simulink model "code_gen"  (Simulink 7.5)
settings: Solver=FixedStepDiscrete  StartTime=0.0  StopTime=10.0  FixedStep=0.001  RelTol=1e-3
InitFcn:
  | boat_constants
values from neighbouring files (symbols this model uses):
  InitialPoint = 0    [boat_constants.m]    (also in l2plus.m)
  IPStar = 0    [boat_constants.m]    (also in l2plus.m)
  ISA_g = 9.815    [boat_constants.m]
  MaxDwnPthStar = 1    [boat_constants.m]    (also in l2plus.m)
  OC2max = 49999    [boat_constants.m]    (also in simulation_constants.m)
  switchDistance = 4    [boat_constants.m]    (also in l2plus.m)
  T_step = 0.01    [boat_constants.m]    (also in common.m)
  tanIntercept = tan( 45*pi/180 )    [boat_constants.m]    (also in l2plus.m)
  TStar = single(4.5)    [boat_constants.m]    (also in l2plus.m = single(2))
  Turn2Track = 0    [boat_constants.m]    (also in l2plus.m)
undefined symbols (not defined in the file or in its folder): buildAndCheckMessage, buildAndCheckSentence, DiscIntNeverNeededParam, ecan1_buffered_transmit_matlab, ecan1_init, getGpsMainData, getSensorData, u1, y1
libraries: simulink x49, dsPICdrivers x22, simulink_need_slupdate x6, microSimulink x4, aerolibconvert2 x3
(part 2 of 3)

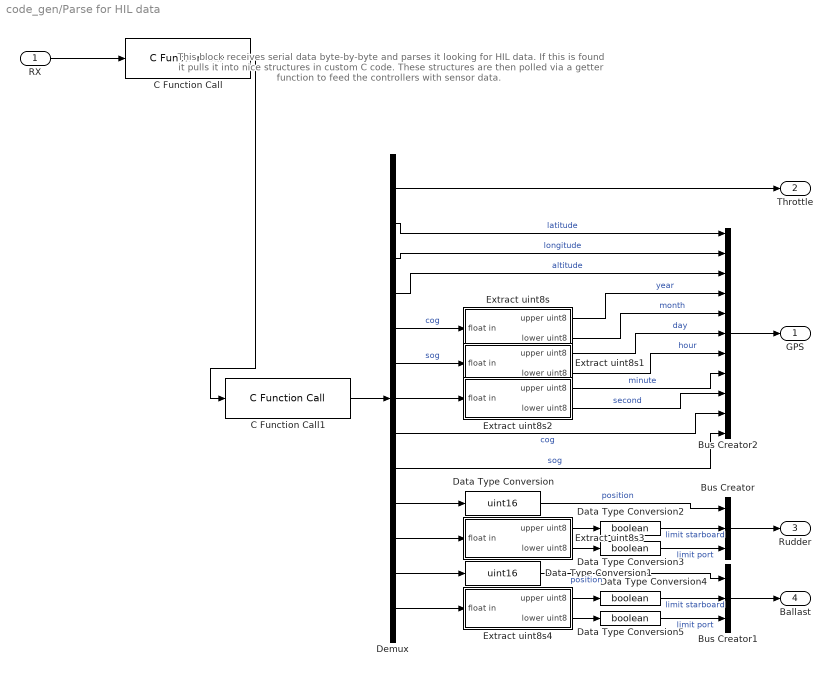
== system code_gen/Parse for HIL data ==
  note: This block receives serial data byte-by-byte and parses it looking for HIL data.
      | If this is found it pulls it into nice structures in custom C code. These structures
      | are then polled via a getter function to feed the controllers with sensor data.
  RX : Inport
  Bus Creator : BusCreator  Inputs=3
  Bus Creator1 : BusCreator  Inputs=3
  Bus Creator2 : BusCreator  Inputs=11
  C Function Call : dsPICdrivers/OTHERS/C Function Call  Tag=dsPIC_dsPIC_CFunctionCall  fctName='buildAndCheckMessage'  INPUT_SIZE=1  INPUT1=uint8  INPUT2=--  INPUT3=--  OUTPUT_SIZE=1  OUTPUT1=--  SampleTime=-1  InputType=[ 2 ]  OutputType=[ ]  FctDeclaration=extern void buildAndCheckMessage(uint8_T u1);  FctCall=buildAndCheckMessage(%u1);  OrderingInOutPopup=Output
  C Function Call1 : dsPICdrivers/OTHERS/C Function Call  Tag=dsPIC_dsPIC_CFunctionCall  fctName='getSensorData'  INPUT_SIZE=1  INPUT1=--  INPUT2=--  INPUT3=--  OUTPUT_SIZE=13  OUTPUT1=real32  SampleTime=.01  InputType=[ ]  OutputType=[ 7 ]  FctDeclaration=extern void getSensorData(real32_T* y1);  FctCall=getSensorData(*%y1);  OrderingInOutPopup=Input
  Data Type Conversion : DataTypeConversion  OutDataTypeMode=uint16  OutDataType=fixdt(1, 16)  OutScaling=2^0  OutDataTypeStr=uint16  ConvertRealWorld=Stored Integer (SI)  RndMeth=Simplest
  Data Type Conversion1 : DataTypeConversion  OutDataTypeMode=uint16  OutDataType=fixdt(1, 16)  OutScaling=2^0  OutDataTypeStr=uint16  ConvertRealWorld=Stored Integer (SI)  RndMeth=Simplest
  Data Type Conversion{2..5} (4 alike) : DataTypeConversion  OutDataTypeMode=boolean  OutDataType=fixdt(1, 16)  OutScaling=2^0  OutDataTypeStr=boolean
  Demux : Demux  Outputs=13
  Extract uint8s : Subsystem
  Extract uint8s1 : Subsystem
  Extract uint8s2 : Subsystem
  Extract uint8s3 : Subsystem
  Extract uint8s4 : Subsystem
  GPS : Outport
  Throttle : Outport  Port=2
  Rudder : Outport  Port=3
  Ballast : Outport  Port=4
  wires:
  RX/1 -> C Function Call/1
  Demux/1 -> Throttle/1
  Bus Creator/1 -> Rudder/1
  Extract uint8s3/1(upper uint8) -> Data Type Conversion2/1
  Demux/10 -> Data Type Conversion/1
  Extract uint8s3/2(lower uint8) -> Data Type Conversion3/1
  Bus Creator1/1 -> Ballast/1
  Extract uint8s4/1(upper uint8) -> Data Type Conversion4/1
  Demux/12 -> Data Type Conversion1/1
  Extract uint8s4/2(lower uint8) -> Data Type Conversion5/1
  Bus Creator2/1 -> GPS/1
  Demux/4 -> Bus Creator2/3  "altitude"
  Demux/3 -> Bus Creator2/2  "longitude"
  Demux/2 -> Bus Creator2/1  "latitude"
  C Function Call1/1 -> Demux/1
  Demux/11 -> Extract uint8s3/1(float in)
  Demux/13 -> Extract uint8s4/1(float in)
  Data Type Conversion/1 -> Bus Creator/1  "position"
  Data Type Conversion1/1 -> Bus Creator1/1  "position"
  Extract uint8s2/2(lower uint8) -> Bus Creator2/9  "second"
  Extract uint8s2/1(upper uint8) -> Bus Creator2/8  "minute"
  Extract uint8s1/2(lower uint8) -> Bus Creator2/7  "hour"
  Extract uint8s1/1(upper uint8) -> Bus Creator2/6  "day"
  Extract uint8s/2(lower uint8) -> Bus Creator2/5  "month"
  Extract uint8s/1(upper uint8) -> Bus Creator2/4  "year"
  Demux/5 -> Extract uint8s/1(float in)  "cog"
  Demux/6 -> Extract uint8s1/1(float in)  "sog"
  Demux/7 -> Extract uint8s2/1(float in)
  Demux/8 -> Bus Creator2/10  "cog"
  Demux/9 -> Bus Creator2/11  "sog"
  Data Type Conversion2/1 -> Bus Creator/2  "limit starboard"
  Data Type Conversion3/1 -> Bus Creator/3  "limit port"
  Data Type Conversion4/1 -> Bus Creator1/2  "limit starboard"
  Data Type Conversion5/1 -> Bus Creator1/3  "limit port"
  C Function Call/1 -> C Function Call1/1

== system code_gen/Propulsion Outputs ==
  note: Propulsion is controlled here via a CAN interface to the motor driver board.
      | ECAN1 is used and several possible commands are transmitted: enable, disable,
      | or change speed, with speed being between -1023 and 1023 taken as a fraction
      | of total speed (1023).
  In1 : Inport  OutDataType=fixdt(1, 16)  OutScaling=2^0
  Bus Selector : BusSelector  OutputSignals=identifier,data,size,trigger
  To Drive Motor : Subsystem  mask(Send ECAN Message){buffer=0, identifier=hex2dec('401'), identifier_from_input=on, ide=off, remote=off, data=[hex2dec('11') hex2dec('12') hex2dec('13') hex2dec('14')], data_length=4, data_from_input=on, c_func_sample_time=.01, trigger_on_input=on}
      mask prompts: identifier_from_input "Identifier from input"; data_length "Data length"; data_from_input "Data from input"; c_func_sample_time "Sample time"; trigger_on_input "Trigger on input"
      mask help: This block allows for the transmission of a message over the ECAN module.
      mask CallbackString:
      | ||mEnables = get_param(gcb,'MaskEnables');
      | enabled = get_param(gcb, 'identifier_from_input');
      | if strcmp(enabled,'on');
      |     replace_block([gcb '/identifier'],'Constant','Inport','noprompt');
      |     mEnables{2} = 'off';
      |     set_param([gcb '/identifier'],'Port','1');
      | else
      |     replace_block([gcb '/identifier'],'Inport','Constant','noprompt');
      |     mEnables{2} = 'on';
      |     set_param([gcb '/identifier'],'Value','identifier');
      | end
      | set_param(gcb, 'MaskEnables', mEnables);
      | |||data = eval(get_param(gcb, 'data'));
      | y = size(data,1);
      | x = size(data,2);
      | if y > 1 && x > 1
      |     error('Data must be a 1-dimensional vector')
      | else
      |     if or(x > 8, y > 8)
      |         error('Data cannot be larger than 8-bytes');
      |     end
      | end
      | 
      | set_param(gcb, 'data_length', num2str(length(data)));|data_length = eval(get_param(gcb, 'data_length'));
      | if or(data_length < 0, data_length > 9)
      |     error('Data cannot be more than 8 bytes or less than 0.')
      | end|mEnables = get_param(gcb,'MaskEnables');
      | enabled = get_param(gcb, 'data_from_input');
      | if strcmp(enabled,'on');
      |     replace_block([gcb '/data'],'Constant','Inport','noprompt');
      |     replace_block([gcb '/data_length'],'Constant','Inport','noprompt');
      |     mEnables{6} = 'off';
      |     mEnables{7} = 'off';
      |     port = 1;
      |     if ~isempty(find_system(gcb,'LookUnderMasks','all','Name','identifier'))
      |         port = 2;
      |     end
      |     set_param([gcb '/data'],'Port',num2str(port));
      |     set_param([gcb '/data_length'],'Port',num2str(port+1));
      | else
      |     replace_block([gcb '/data'],'Inport','Constant','noprompt');
      |     replace_block([gcb '/data_length'],'Inport','Constant','noprompt');
      |     mEnables{6} = 'on';
      |     mEnables{7} = 'on';
      |     set_param([gcb '/data'],'Value','data');
      |     set_param([gcb '/data'],'OutDataTypeMode','uint8');
      |     set_param([gcb '/data_length'],'Value','data_length');
      |     set_param([gcb '/data_length'],'OutDataTypeMode','uint8');
      | end
      | set_param(gcb, 'MaskEnables', mEnables);
      | ||mEnables = get_param(gcb,'MaskEnables');
      | enabled = get_param(gcb, 'trigger_on_input');
      | c_func_blk = find_system(gcb,'LookUnderMasks','all','FunctionName','dsPIC_C_function_Call');
      | if strcmp(enabled,'on');
      |     mEnables{9} = 'off';
      |     %set_param(c_func_blk,'SampleTime','-1');
      |     replace_block([gcb '/trigger'],'Constant','Inport','noprompt');
      | else
      |     mEnables{9} = 'on';
      |     %set_param(c_func_blk,'SampleTime','c_func_sample_time');
      |     replace_block([gcb '/trigger'],'Inport','Constant','noprompt');
      |     %set_param([gcb '/trigger'],'Value','1');
      | end
      | set_param(gcb, 'MaskEnables', mEnables);
      mask Display: disp('ECAN1 TX');
  wires:
  In1/1 -> Bus Selector/1
  Bus Selector/1 -> To Drive Motor/1(identifier)  "<identifier>"
  Bus Selector/2 -> To Drive Motor/2(data)  "<data>"
  Bus Selector/3 -> To Drive Motor/3(data_length)  "<size>"
  Bus Selector/4 -> To Drive Motor/4(trigger)  "<trigger>"

== system code_gen/Radio Control Inputs ==
  note: IC2 is used to control the reset as the throttle has a heartbeat PWM output upon disconnect.
      | Every other channel will be disabled with no pulses, so anything besides the throttle channel
      | should work fine.
  Clear to Zero if Disconnect : Subsystem
  Compare To Constant : simulink/Logic and Bit Operations/Compare To Constant  SystemSampleTime=-1  relop=>  const=7500  LogicOutDataTypeMode=boolean
  RC Input : dsPICdrivers/Peripheral I//O/Input Capture  Tag=dsPIC_PWM_IC  Priority=5  IntPriority=7  Channel=[2 3 4]  Channel_UP_Down_Periode="[1  1  1]"  MaxChannel="[0.002       0.002       0.002]"  SafeMarge="[10  10  10]"  MaxName=' IC2max , IC3max , IC4max '  Precision="[13.425       13.425       13.425]"  Timer="[2  2  2]"  ChangeDetected="[2  2  2]"  ChangeDetectedPortRef=3  SampleTime=.1  Status=OK
  Rate Transition : RateTransition
  Rate Transition1 : RateTransition
  Rate Transition2 : RateTransition
  Terminator1 : Terminator
  Terminator2 : Terminator
  Rudder : Outport
  Throttle : Outport  Port=2
  Mode : Outport  Port=3
  wires:
  Clear to Zero if Disconnect/2(o2) -> Rate Transition1/1
  Clear to Zero if Disconnect/1(o1) -> Rate Transition/1
  Clear to Zero if Disconnect/3(o3) -> Rate Transition2/1
  RC Input/1 -> Clear to Zero if Disconnect/2(ch1)
  RC Input/3 -> Clear to Zero if Disconnect/3(ch2)
  RC Input/5 -> Clear to Zero if Disconnect/4(ch3)
  Rate Transition/1 -> Rudder/1
  Rate Transition1/1 -> Throttle/1
  Rate Transition2/1 -> Compare To Constant/1
  RC Input/2 -> Clear to Zero if Disconnect/1(Reset)
  RC Input/6 -> Terminator1/1
  Compare To Constant/1 -> Mode/1
  RC Input/4 -> Terminator2/1

== system code_gen/Rudder Outputs ==
  note: Rudder commands are output via a pulse-train signaling step (through the OC2 pins),
      | a direction bit set via RD5, and an enable bit set via RG9.
  In1 : Inport
  Bus Selector : BusSelector  OutputSignals=enable,direction,up,period
  Digital Output Write : dsPICdrivers/Digital I//O/Digital Output Write  Tag=dsPIC_Digital_Output  Priority=5  PORT=D  Pin=[5]  Simultaneous=off  OrderingInOutPopup=None
  Digital Output Write1 : dsPICdrivers/Digital I//O/Digital Output Write  Tag=dsPIC_Digital_Output  Priority=5  PORT=G  Pin=[9]  Simultaneous=off  OrderingInOutPopup=None
  Rudder Motor : dsPICdrivers/Peripheral I//O/Output Compare  Tag=dsPIC_PWM_out  Priority=5  IntPriority=3  CHANNEL=[2]  Channel_UP_Down_Periode=[5]  MaxChannel=[0.01]  MaxName=' OC2max '  Precision=[15.6096]  Timer=[2]  Status=OK  SafeMarge=[0]  PortLetter=[68]  PortNumber=[1]  MaxValues=[49999]
  wires:
  Bus Selector/2 -> Digital Output Write/1  "<direction>"
  Bus Selector/1 -> Digital Output Write1/1  "<enable>"
  Bus Selector/3 -> Rudder Motor/1  "<up>"
  Bus Selector/4 -> Rudder Motor/2  "<period>"
  In1/1 -> Bus Selector/1

== system code_gen/Rudder Sensors ==
  note: The rudder has two main sensors: hall effect and a potentiometer. The
      | potentiometer returns a voltage value through the onboard ADC indicating
      | rudder position exactly. The three Hall effect sensors are used as limit switches
      | indicating port and starboard limits as well as center, though this sensor isn't
      | being used currently.
      |
      | It expects a range of 1.12-2.11V for the rudder position potentiometer with
      | 2.11V being hard to port. The potentiometer was powered at 3.3V for these
      | measurements.
  Bus Creator : BusCreator  Inputs=3
  Port Hall : dsPICdrivers/Digital I//O/Digital Input  Tag=dsPIC_Digital_Input  PORT=F  Pin=[3]  SampleTime=.01  OrderingInOutPopup=None
  Rudder Potentiometer : dsPICdrivers/Peripheral I//O/ADC Input  Tag=dsPIC_ADC  Priority=5  ADC_TYPE=10 bits  ADC_MODE=Continuous sampling & get last channel value  NbrSampleStep=1  VoltRefpopup="AVdd  -  AVss"  OutFormatBitspopup=ssss sssd dddd dddd : Signed Integer  InterruptPriority=6  ANCHANNELS=[0]  MaxName=ANmax = 1023  Rin=1e2  ADCS=12  SAMC=1  Temperature=25  DMAChannel=7  SampleTime=.01  Status="OK  |  Tsmp=1.625e-007 |  T/Channel=2.113e-006 |  Tall=2.113e-006"  SSRC=auto convert
  Starboard Hall : dsPICdrivers/Digital I//O/Digital Input  Tag=dsPIC_Digital_Input  PORT=G  Pin=[3]  SampleTime=.01  OrderingInOutPopup=None
  Out1 : Outport
  wires:
  Rudder Potentiometer/1 -> Bus Creator/1  "position"
  Starboard Hall/1 -> Bus Creator/2  "limit starboard"
  Port Hall/1 -> Bus Creator/3  "limit port"
  Bus Creator/1 -> Out1/1

== system code_gen/Throttle Command ==
  sensors : Inport
  speed : Inport  Port=2
  Bus Creator : BusCreator
  Mux Everything : Subsystem
  Terminator : Terminator
  Trigger Events : Subsystem
  command : Outport  OutDataType=sfix(16)  OutScaling=2^0
  wires:
  sensors/1 -> Terminator/1
  Bus Creator/1 -> command/1
  Trigger Events/1(Change Speed) -> Mux Everything/1(speed)
  Trigger Events/3(Enable) -> Mux Everything/3(enable)
  Trigger Events/2(Disable) -> Mux Everything/2(disable)
  speed/1 -> Mux Everything/4(Throttle), Trigger Events/1(RC Throttle)
  Mux Everything/1(iden) -> Bus Creator/1  "identifier"
  Mux Everything/2(data) -> Bus Creator/2  "data"
  Mux Everything/3(size) -> Bus Creator/3  "size"
  Mux Everything/4(trig) -> Bus Creator/4  "trigger"

== system code_gen/Throttle Sensors ==
  note: Throttle output is currently being ignored. The motor driver board
      | should report current velocity along with other status information
      | on a regular basis and that could be parsed for this information. As
      | of right now it's been deemed non-critical and therefore ignored.
  Constant : Constant  Value=0  OutDataType=fixdt(1, 16)  OutScaling=2^0  SampleTime=.01
  Out1 : Outport
  wires:
  Constant/1 -> Out1/1

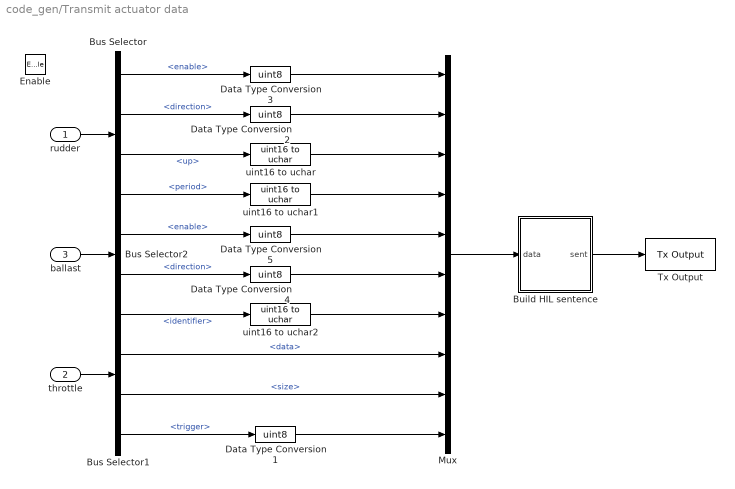
== system code_gen/Transmit actuator data ==
  rudder : Inport  OutDataType=fixdt(1, 16)  OutScaling=2^0
  throttle : Inport  Port=2  OutDataType=fixdt(1, 16)  OutScaling=2^0
  ballast : Inport  Port=3  OutDataType=fixdt(1, 16)  OutScaling=2^0
  Enable : EnablePort
  Build HIL sentence : Subsystem
  Bus Selector : BusSelector  OutputSignals=enable,direction,up,period
  Bus Selector1 : BusSelector  OutputSignals=identifier,data,size,trigger
  Bus Selector2 : BusSelector  OutputSignals=enable,direction
  Data Type Conversion{1..5} (5 alike) : DataTypeConversion  OutDataTypeMode=uint8  OutDataType=fixdt(1, 16)  OutScaling=2^0  OutDataTypeStr=uint8
  Mux : Mux  Inputs=10
  Tx Output : dsPICdrivers/Serial PORT/Tx Output  Tag=dsPIC_TX  Priority=5  UART=2  OrderingInOutPopup=None
  uint16 to uchar : microSimulink/Conversions/uint16 to uchar  SystemSampleTime=-1
  uint16 to uchar1 : microSimulink/Conversions/uint16 to uchar  SystemSampleTime=-1
  uint16 to uchar2 : microSimulink/Conversions/uint16 to uchar  SystemSampleTime=-1
  wires:
  rudder/1 -> Bus Selector/1
  Bus Selector/2 -> Data Type Conversion2/1  "<direction>"
  Bus Selector/1 -> Data Type Conversion3/1  "<enable>"
  throttle/1 -> Bus Selector1/1
  Bus Selector1/4 -> Data Type Conversion1/1  "<trigger>"
  Data Type Conversion2/1 -> Mux/2
  Bus Selector1/3 -> Mux/9  "<size>"
  Bus Selector1/1 -> uint16 to uchar2/1  "<identifier>"
  Data Type Conversion1/1 -> Mux/10
  Build HIL sentence/1(sent) -> Tx Output/1
  Mux/1 -> Build HIL sentence/1(data)
  Data Type Conversion3/1 -> Mux/1
  Bus Selector/3 -> uint16 to uchar/1  "<up>"
  ballast/1 -> Bus Selector2/1
  Bus Selector2/1 -> Data Type Conversion5/1  "<enable>"
  Bus Selector2/2 -> Data Type Conversion4/1  "<direction>"
  Bus Selector/4 -> uint16 to uchar1/1  "<period>"
  uint16 to uchar/1 -> Mux/3
  uint16 to uchar1/1 -> Mux/4
  uint16 to uchar2/1 -> Mux/7
  Bus Selector1/2 -> Mux/8  "<data>"
  Data Type Conversion4/1 -> Mux/6
  Data Type Conversion5/1 -> Mux/5

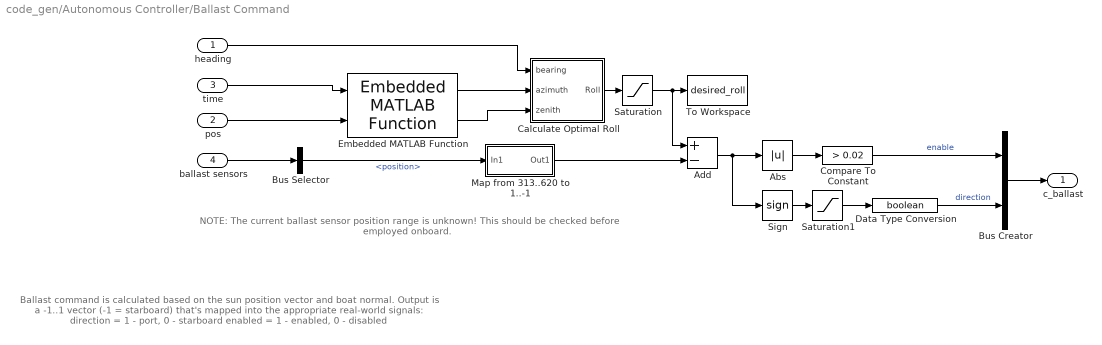
== system code_gen/Autonomous Controller/Ballast Command ==
  note: Ballast command is calculated based on the sun position vector
      | and boat normal. Output is a -1..1 vector (-1 = starboard) that's
      |  mapped into the appropriate real-world signals:
      | direction = 1 - port, 0 - starboard
      | enabled = 1 - enabled, 0 - disabled
  note: NOTE: The current ballast sensor position range is
      | unknown! This should be checked before employed
      | onboard.
  heading : Inport
  pos : Inport  Port=2
  time : Inport  Port=3
  ballast sensors : Inport  Port=4
  Abs : Abs  OutDataType=fixdt(1, 16)  OutScaling=2^0
  Add : Sum  Inputs=+-  OutDataType=fixdt(1, 16)  OutScaling=2^-10
  Bus Creator : BusCreator  Inputs=2
  Bus Selector : BusSelector  OutputSignals=position
  Calculate Optimal Roll : Subsystem
  Compare To Constant : simulink/Logic and Bit Operations/Compare To Constant  SystemSampleTime=-1  relop=>  const=0.02  LogicOutDataTypeMode=boolean
  Data Type Conversion : DataTypeConversion  OutDataTypeMode=boolean  OutDataType=fixdt(1, 16)  OutScaling=2^0  OutDataTypeStr=boolean  RndMeth=Simplest
  Embedded MATLAB Function : microSimulink/Embedded MATLAB Function  SystemSampleTime=-1
  Map from 313..620 to 1..-1 : Subsystem
  Saturation : Saturate  UpperLimit=1  LowerLimit=-1
  Saturation1 : Saturate  UpperLimit=1  LowerLimit=0  OutDataTypeStr=Inherit: Inherit via back propagation
  Sign : Signum
  To Workspace : ToWorkspace  VariableName=desired_roll  SampleTime=-1  SaveFormat=Structure
  c_ballast : Outport
  wires:
  Data Type Conversion/1 -> Bus Creator/2  "direction"
  Calculate Optimal Roll/1(Roll) -> Saturation/1
  time/1 -> Embedded MATLAB Function/1
  Bus Creator/1 -> c_ballast/1
  ballast sensors/1 -> Bus Selector/1
  Bus Selector/1 -> Map from 313..620 to 1..-1/1(In1)  "<position>"
  Saturation/1 -> Add/1, To Workspace/1
  Add/1 -> Abs/1, Sign/1
  Sign/1 -> Saturation1/1
  Abs/1 -> Compare To Constant/1
  Compare To Constant/1 -> Bus Creator/1  "enable"
  Saturation1/1 -> Data Type Conversion/1
  pos/1 -> Embedded MATLAB Function/2
  heading/1 -> Calculate Optimal Roll/1(bearing)
  Embedded MATLAB Function/1 -> Calculate Optimal Roll/2(azimuth)
  Embedded MATLAB Function/2 -> Calculate Optimal Roll/3(zenith)
  Map from 313..620 to 1..-1/1(Out1) -> Add/2

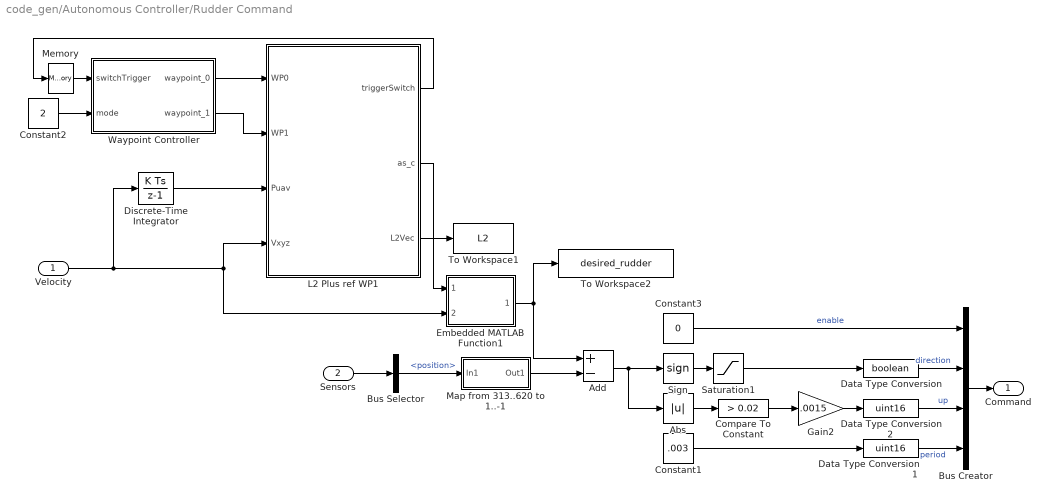
== system code_gen/Autonomous Controller/Rudder Command ==
  Velocity : Inport
  Sensors : Inport  Port=2
  Abs : Abs  OutDataType=fixdt(1, 16)  OutScaling=2^0
  Add : Sum  Inputs=+-  OutDataType=fixdt(1, 16)  OutScaling=2^-10
  Bus Creator : BusCreator
  Bus Selector : BusSelector  OutputSignals=position
  Compare To Constant : simulink/Logic and Bit Operations/Compare To Constant  SystemSampleTime=-1  relop=>  const=0.02  LogicOutDataTypeMode=uint8
  Constant1 : Constant  Value=.003  OutDataTypeMode=single  OutDataType=sfix(16)  OutScaling=2^0  OutDataTypeStr=single
  Constant2 : Constant  Value=2  OutDataTypeMode=uint8  OutDataType=sfix(16)  OutScaling=2^0  OutDataTypeStr=uint8
  Constant3 : Constant  Value=0  OutDataTypeMode=boolean  OutDataType=sfix(16)  OutScaling=2^0  OutDataTypeStr=boolean
  Data Type Conversion : DataTypeConversion  OutDataTypeMode=boolean  OutDataType=fixdt(1, 16)  OutScaling=2^0  OutDataTypeStr=boolean  RndMeth=Simplest
  Data Type Conversion1 : DataTypeConversion  OutDataTypeMode=uint16  OutDataType=fixdt(1, 16)  OutScaling=2^0  OutDataTypeStr=uint16  RndMeth=Simplest
  Data Type Conversion2 : DataTypeConversion  OutDataTypeMode=uint16  OutDataType=fixdt(1, 16)  OutScaling=2^0  OutDataTypeStr=uint16  RndMeth=Simplest
  Discrete-Time Integrator : DiscreteIntegrator  InitialConditionMode=State only (most efficient)  SampleTime=T_step  OutDataType=fixdt(1, 16)  OutScaling=2^0  ICPrevOutput=DiscIntNeverNeededParam  ICPrevScaledInput=DiscIntNeverNeededParam
  Embedded MATLAB Function1 : Stateflow chart  TreatAsAtomicUnit=on
  Gain2 : Gain  Gain=.0015  ParameterDataType=sfix(16)  ParameterScaling=2^0  OutDataTypeMode=single  OutDataType=sfix(16)  OutScaling=2^0  OutDataTypeStr=single
  L2 Plus ref WP1 : Stateflow chart  TreatAsAtomicUnit=on  SystemSampleTime=.01
  Map from 313..620 to 1..-1 : Subsystem
  Memory : Memory  InheritSampleTime=on
  Saturation1 : Saturate  UpperLimit=1  LowerLimit=0  OutDataTypeStr=Inherit: Inherit via back propagation
  Sign : Signum
  To Workspace1 : ToWorkspace  VariableName=L2  SampleTime=-1  SaveFormat=Array
  To Workspace2 : ToWorkspace  VariableName=desired_rudder  SampleTime=-1  SaveFormat=Array
  Waypoint Controller : Stateflow chart  TreatAsAtomicUnit=on
      settings: MinAlgLoopOccurrences=on
  Command : Outport
  wires:
  Constant3/1 -> Bus Creator/1  "enable"
  Data Type Conversion2/1 -> Bus Creator/3  "up"
  Data Type Conversion1/1 -> Bus Creator/4  "period"
  L2 Plus ref WP1/2(as_c) -> Embedded MATLAB Function1/1(lat_accel)
  Velocity/1 -> L2 Plus ref WP1/4(Vxyz), Embedded MATLAB Function1/2(velocity), Discrete-Time Integrator/1
  L2 Plus ref WP1/3(L2Vec) -> To Workspace1/1
  Waypoint Controller/2(waypoint_1) -> L2 Plus ref WP1/2(WP1)
  Waypoint Controller/1(waypoint_0) -> L2 Plus ref WP1/1(WP0)
  L2 Plus ref WP1/1(triggerSwitch) -> Memory/1
  Constant2/1 -> Waypoint Controller/2(mode)
  Memory/1 -> Waypoint Controller/1(switchTrigger)
  Embedded MATLAB Function1/1(rudder) -> To Workspace2/1, Add/1
  Add/1 -> Abs/1, Sign/1
  Sign/1 -> Saturation1/1
  Abs/1 -> Compare To Constant/1
  Compare To Constant/1 -> Gain2/1
  Saturation1/1 -> Data Type Conversion/1
  Gain2/1 -> Data Type Conversion2/1
  Constant1/1 -> Data Type Conversion1/1
  Bus Creator/1 -> Command/1
  Sensors/1 -> Bus Selector/1
  Discrete-Time Integrator/1 -> L2 Plus ref WP1/3(Puav)
  Map from 313..620 to 1..-1/1(Out1) -> Add/2
  Bus Selector/1 -> Map from 313..620 to 1..-1/1(In1)  "<position>"
  Data Type Conversion/1 -> Bus Creator/2  "direction"

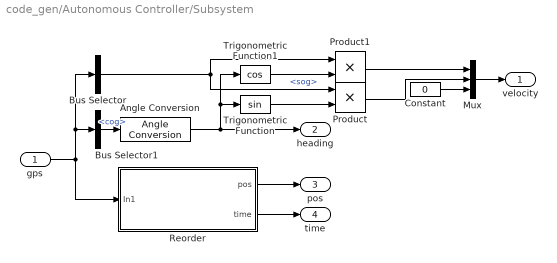
== system code_gen/Autonomous Controller/Subsystem ==
  gps : Inport
  Angle Conversion : aerolibconvert2/Angle Conversion  SystemSampleTime=-1  IU=deg  OU=rad
  Bus Selector : BusSelector  OutputSignals=sog
  Bus Selector1 : BusSelector  OutputSignals=cog
  Constant : Constant  Value=0  OutDataTypeMode=single  OutDataType=fixdt(1, 16)  OutScaling=2^0  OutDataTypeStr=single
  Mux : Mux  Inputs=3
  Product : Product  OutDataTypeMode=single  OutDataType=fixdt(1, 16)  OutScaling=2^0  OutDataTypeStr=single  RndMeth=Zero
  Product1 : Product  OutDataTypeMode=single  OutDataType=fixdt(1, 16)  OutScaling=2^0  OutDataTypeStr=single  RndMeth=Zero
  Reorder : Subsystem
  Trigonometric Function : Trigonometry
  Trigonometric Function1 : Trigonometry  Operator=cos
  velocity : Outport
  heading : Outport  Port=2
  pos : Outport  Port=3
  time : Outport  Port=4
  wires:
  gps/1 -> Bus Selector/1, Bus Selector1/1, Reorder/1(In1)
  Bus Selector1/1 -> Angle Conversion/1  "<cog>"
  Trigonometric Function/1 -> Product/2
  Trigonometric Function1/1 -> Product1/2
  Product1/1 -> Mux/1
  Product/1 -> Mux/2
  Constant/1 -> Mux/3
  Mux/1 -> velocity/1
  Angle Conversion/1 -> heading/1, Trigonometric Function/1, Trigonometric Function1/1
  Bus Selector/1 -> Product1/1, Product/1  "<sog>"
  Reorder/1(pos) -> pos/1
  Reorder/2(time) -> time/1

== system code_gen/Autonomous Controller/Throttle Command ==
  sensors : Inport
  speed : Inport  Port=2
  Bus Creator : BusCreator
  Mux Everything : Subsystem
  Terminator : Terminator
  Trigger Events : Subsystem
  command : Outport  OutDataType=sfix(16)  OutScaling=2^0
  wires:
  Mux Everything/4(trig) -> Bus Creator/4  "trigger"
  Mux Everything/3(size) -> Bus Creator/3  "size"
  Mux Everything/2(data) -> Bus Creator/2  "data"
  Mux Everything/1(iden) -> Bus Creator/1  "identifier"
  speed/1 -> Trigger Events/1(RC Throttle), Mux Everything/4(Throttle)
  Trigger Events/2(Disable) -> Mux Everything/2(disable)
  Trigger Events/3(Enable) -> Mux Everything/3(enable)
  Trigger Events/1(Change Speed) -> Mux Everything/1(speed)
  Bus Creator/1 -> command/1
  sensors/1 -> Terminator/1

== system code_gen/Manual Rudder Command/Map position  into -1024..1023 ==
  input : Inport  OutDataType=sfix(16)  OutScaling=2^0
  Saturation : Saturate  UpperLimit=1023  LowerLimit=-1024
  Weighted Moving Average1 : simulink_need_slupdate/Weighted Moving Average  mgainval=[.5 .5]  vinit=0.0  samptime=-1  OutDataTypeStr=Inherit: Inherit via back propagation  OutDataType=sfix(16)  OutScaling=2^-10  DoSatur=off  GainDataType=uint(16)  MatRadixGroup=Best Precision: Matrix-wise  GainScaling=2^-10
  mapped : Outport  OutDataType=sfix(16)  OutScaling=2^0
  wires:
  Saturation/1 -> Weighted Moving Average1/1
  input/1 -> Saturation/1
  Weighted Moving Average1/1 -> mapped/1

== system code_gen/Manual Rudder Command/Map throttle into -1023..1023 ==
  in : Inport  OutDataType=sfix(16)  OutScaling=2^0
  Bias1 : Bias  Bias=-7215
  Data Type Conversion : DataTypeConversion  OutDataTypeMode=int32  OutDataType=sfix(16)  OutScaling=2^0  OutDataTypeStr=int32
  Data Type Conversion2 : DataTypeConversion  OutDataTypeMode=int16  OutDataType=sfix(16)  OutScaling=2^0  OutDataTypeStr=int16
  Saturation2 : Saturate  UpperLimit=1023  LowerLimit=-1023
  Shift Arithmetic : simulink/Logic and Bit Operations/Shift Arithmetic  SystemSampleTime=-1  nBitShiftRight=10  nBinPtShiftRight=0
  Weighted Moving Average : simulink_need_slupdate/Weighted Moving Average  mgainval=[.2 .2 .2 .2 .2]  vinit=0.0  samptime=-1  OutDataTypeStr=Inherit: Inherit via back propagation  OutDataType=sfix(16)  OutScaling=2^-10  DoSatur=off  GainDataType=uint(16)  MatRadixGroup=Best Precision: Matrix-wise  GainScaling=2^-10
  out : Outport  OutDataType=sfix(16)  OutScaling=2^0
  wires:
  Saturation2/1 -> Weighted Moving Average/1
  Weighted Moving Average/1 -> out/1
  Data Type Conversion2/1 -> Saturation2/1
  Bias1/1 -> Shift Arithmetic/1
  Data Type Conversion/1 -> Bias1/1
  Shift Arithmetic/1 -> Data Type Conversion2/1
  in/1 -> Data Type Conversion/1

== system code_gen/Parse for HIL data/Extract uint8s ==
  float in : Inport
  Data Type Conversion : DataTypeConversion  OutDataTypeMode=uint32  OutDataType=fixdt(1, 16)  OutScaling=2^0  OutDataTypeStr=uint32  ConvertRealWorld=Stored Integer (SI)  RndMeth=Simplest
  Data Type Conversion2 : DataTypeConversion  OutDataTypeMode=uint8  OutDataType=fixdt(1, 16)  OutScaling=2^0  OutDataTypeStr=uint8
  Data Type Conversion3 : DataTypeConversion  OutDataTypeMode=uint8  OutDataType=fixdt(1, 16)  OutScaling=2^0  OutDataTypeStr=uint8
  Extract Bits : simulink/Logic and Bit Operations/Extract Bits  SystemSampleTime=-1  bitsToExtract=Upper half  numBits=8  bitIdxRange=[0 7]  outScalingMode=Treat bit field as an integer
  Extract Bits1 : simulink/Logic and Bit Operations/Extract Bits  SystemSampleTime=-1  bitsToExtract=Lower half  numBits=8  bitIdxRange=[0 7]  outScalingMode=Treat bit field as an integer
  upper uint8 : Outport
  lower uint8 : Outport  Port=2
  wires:
  Data Type Conversion/1 -> Extract Bits/1, Extract Bits1/1
  Extract Bits/1 -> Data Type Conversion2/1
  float in/1 -> Data Type Conversion/1
  Extract Bits1/1 -> Data Type Conversion3/1
  Data Type Conversion2/1 -> upper uint8/1
  Data Type Conversion3/1 -> lower uint8/1

== system code_gen/Parse for HIL data/Extract uint8s1 ==
  float in : Inport
  Data Type Conversion : DataTypeConversion  OutDataTypeMode=uint32  OutDataType=fixdt(1, 16)  OutScaling=2^0  OutDataTypeStr=uint32  ConvertRealWorld=Stored Integer (SI)  RndMeth=Simplest
  Data Type Conversion2 : DataTypeConversion  OutDataTypeMode=uint8  OutDataType=fixdt(1, 16)  OutScaling=2^0  OutDataTypeStr=uint8
  Data Type Conversion3 : DataTypeConversion  OutDataTypeMode=uint8  OutDataType=fixdt(1, 16)  OutScaling=2^0  OutDataTypeStr=uint8
  Extract Bits : simulink/Logic and Bit Operations/Extract Bits  SystemSampleTime=-1  bitsToExtract=Upper half  numBits=8  bitIdxRange=[0 7]  outScalingMode=Treat bit field as an integer
  Extract Bits1 : simulink/Logic and Bit Operations/Extract Bits  SystemSampleTime=-1  bitsToExtract=Lower half  numBits=8  bitIdxRange=[0 7]  outScalingMode=Treat bit field as an integer
  upper uint8 : Outport
  lower uint8 : Outport  Port=2
  wires:
  Data Type Conversion3/1 -> lower uint8/1
  Data Type Conversion2/1 -> upper uint8/1
  Extract Bits1/1 -> Data Type Conversion3/1
  float in/1 -> Data Type Conversion/1
  Extract Bits/1 -> Data Type Conversion2/1
  Data Type Conversion/1 -> Extract Bits1/1, Extract Bits/1

== system code_gen/Parse for HIL data/Extract uint8s2 ==
  float in : Inport
  Data Type Conversion : DataTypeConversion  OutDataTypeMode=uint32  OutDataType=fixdt(1, 16)  OutScaling=2^0  OutDataTypeStr=uint32  ConvertRealWorld=Stored Integer (SI)  RndMeth=Simplest
  Data Type Conversion2 : DataTypeConversion  OutDataTypeMode=uint8  OutDataType=fixdt(1, 16)  OutScaling=2^0  OutDataTypeStr=uint8
  Data Type Conversion3 : DataTypeConversion  OutDataTypeMode=uint8  OutDataType=fixdt(1, 16)  OutScaling=2^0  OutDataTypeStr=uint8
  Extract Bits : simulink/Logic and Bit Operations/Extract Bits  SystemSampleTime=-1  bitsToExtract=Upper half  numBits=8  bitIdxRange=[0 7]  outScalingMode=Treat bit field as an integer
  Extract Bits1 : simulink/Logic and Bit Operations/Extract Bits  SystemSampleTime=-1  bitsToExtract=Lower half  numBits=8  bitIdxRange=[0 7]  outScalingMode=Treat bit field as an integer
  upper uint8 : Outport
  lower uint8 : Outport  Port=2
  wires:
  Data Type Conversion/1 -> Extract Bits/1, Extract Bits1/1
  Extract Bits/1 -> Data Type Conversion2/1
  float in/1 -> Data Type Conversion/1
  Extract Bits1/1 -> Data Type Conversion3/1
  Data Type Conversion2/1 -> upper uint8/1
  Data Type Conversion3/1 -> lower uint8/1

== system code_gen/Parse for HIL data/Extract uint8s3 ==
  float in : Inport
  Data Type Conversion : DataTypeConversion  OutDataTypeMode=uint32  OutDataType=fixdt(1, 16)  OutScaling=2^0  OutDataTypeStr=uint32  ConvertRealWorld=Stored Integer (SI)  RndMeth=Simplest
  Data Type Conversion2 : DataTypeConversion  OutDataTypeMode=uint8  OutDataType=fixdt(1, 16)  OutScaling=2^0  OutDataTypeStr=uint8
  Data Type Conversion3 : DataTypeConversion  OutDataTypeMode=uint8  OutDataType=fixdt(1, 16)  OutScaling=2^0  OutDataTypeStr=uint8
  Extract Bits : simulink/Logic and Bit Operations/Extract Bits  SystemSampleTime=-1  bitsToExtract=Upper half  numBits=8  bitIdxRange=[0 7]  outScalingMode=Treat bit field as an integer
  Extract Bits1 : simulink/Logic and Bit Operations/Extract Bits  SystemSampleTime=-1  bitsToExtract=Lower half  numBits=8  bitIdxRange=[0 7]  outScalingMode=Treat bit field as an integer
  upper uint8 : Outport
  lower uint8 : Outport  Port=2
  wires:
  Data Type Conversion3/1 -> lower uint8/1
  Data Type Conversion2/1 -> upper uint8/1
  Extract Bits1/1 -> Data Type Conversion3/1
  float in/1 -> Data Type Conversion/1
  Extract Bits/1 -> Data Type Conversion2/1
  Data Type Conversion/1 -> Extract Bits1/1, Extract Bits/1

== system code_gen/Parse for HIL data/Extract uint8s4 ==
  float in : Inport
  Data Type Conversion : DataTypeConversion  OutDataTypeMode=uint32  OutDataType=fixdt(1, 16)  OutScaling=2^0  OutDataTypeStr=uint32  ConvertRealWorld=Stored Integer (SI)  RndMeth=Simplest
  Data Type Conversion2 : DataTypeConversion  OutDataTypeMode=uint8  OutDataType=fixdt(1, 16)  OutScaling=2^0  OutDataTypeStr=uint8
  Data Type Conversion3 : DataTypeConversion  OutDataTypeMode=uint8  OutDataType=fixdt(1, 16)  OutScaling=2^0  OutDataTypeStr=uint8
  Extract Bits : simulink/Logic and Bit Operations/Extract Bits  SystemSampleTime=-1  bitsToExtract=Upper half  numBits=8  bitIdxRange=[0 7]  outScalingMode=Treat bit field as an integer
  Extract Bits1 : simulink/Logic and Bit Operations/Extract Bits  SystemSampleTime=-1  bitsToExtract=Lower half  numBits=8  bitIdxRange=[0 7]  outScalingMode=Treat bit field as an integer
  upper uint8 : Outport
  lower uint8 : Outport  Port=2
  wires:
  Data Type Conversion/1 -> Extract Bits/1, Extract Bits1/1
  Extract Bits/1 -> Data Type Conversion2/1
  float in/1 -> Data Type Conversion/1
  Extract Bits1/1 -> Data Type Conversion3/1
  Data Type Conversion2/1 -> upper uint8/1
  Data Type Conversion3/1 -> lower uint8/1

== system code_gen/Propulsion Outputs/To Drive Motor ==
  identifier : Inport  OutDataType=sfix(16)  OutScaling=2^0
  data : Inport  Port=2  OutDataType=sfix(16)  OutScaling=2^0
  data_length : Inport  Port=3  OutDataType=sfix(16)  OutScaling=2^0
  trigger : Inport  Port=4
  C-function Call : Subsystem
  Constant : Constant  Value=buffer  OutDataTypeMode=uint8  OutDataType=sfix(16)  OutScaling=2^0  OutDataTypeStr=uint8
  Constant2 : Constant  Value=ide  OutDataTypeMode=uint8  OutDataType=sfix(16)  OutScaling=2^0  OutDataTypeStr=uint8
  Constant3 : Constant  Value=remote  OutDataTypeMode=uint8  OutDataType=sfix(16)  OutScaling=2^0  OutDataTypeStr=uint8
  Extract Bits : simulink/Logic and Bit Operations/Extract Bits  SystemSampleTime=-1  bitsToExtract=Upper half  numBits=8  bitIdxRange=[0 7]  outScalingMode=Treat bit field as an integer
  Extract Bits1 : simulink/Logic and Bit Operations/Extract Bits  SystemSampleTime=-1  bitsToExtract=Lower half  numBits=8  bitIdxRange=[0 7]  outScalingMode=Preserve fixed-point scaling
  myMux : Stateflow chart  TreatAsAtomicUnit=on
  uint8 combiner1 : Subsystem
  uint8 combiner2 : Subsystem
  wires:
  trigger/1 -> C-function Call/Enable
  myMux/1(y) -> C-function Call/1(parameters)
  uint8 combiner2/1(combined) -> myMux/1(u1)
  Constant/1 -> uint8 combiner2/1(high-order)
  data_length/1 -> uint8 combiner2/2(low-order)
  Extract Bits/1 -> myMux/3(u3)
  Extract Bits1/1 -> myMux/2(u2)
  identifier/1 -> Extract Bits1/1, Extract Bits/1
  uint8 combiner1/1(combined) -> myMux/4(u4)
  Constant3/1 -> uint8 combiner1/2(low-order)
  Constant2/1 -> uint8 combiner1/1(high-order)
  data/1 -> myMux/5(u5)

== system code_gen/Radio Control Inputs/Clear to Zero if Disconnect ==
  Reset : Inport  OutDataType=sfix(16)  OutScaling=2^0
  ch1 : Inport  Port=2  OutDataType=sfix(16)  OutScaling=2^0
  ch2 : Inport  Port=3  OutDataType=sfix(16)  OutScaling=2^0
  ch3 : Inport  Port=4  OutDataType=sfix(16)  OutScaling=2^0
  Constant : Constant  Value=0  OutDataTypeMode=uint16  OutDataType=sfix(16)  OutScaling=2^0  OutDataTypeStr=uint16
  Constant1 : Constant  OutDataTypeMode=uint16  OutDataType=sfix(16)  OutScaling=2^0  OutDataTypeStr=uint16
  Discrete-Time Integrator : DiscreteIntegrator  IntegratorMethod=Accumulation: Forward Euler  ExternalReset=level  InitialConditionMode=State only (most efficient)  SampleTime=-1  OutDataType=sfix(16)  OutScaling=2^0  LimitOutput=on  UpperSaturationLimit=50  LowerSaturationLimit=0  ICPrevOutput=DiscIntNeverNeededParam  ICPrevScaledInput=DiscIntNeverNeededParam
  Switch : Switch  Criteria=u2 > Threshold  Threshold=40
  Switch1 : Switch  Criteria=u2 > Threshold  Threshold=40
  Switch2 : Switch  Criteria=u2 > Threshold  Threshold=40
  o1 : Outport  OutDataType=sfix(16)  OutScaling=2^0
  o2 : Outport  Port=2  OutDataType=sfix(16)  OutScaling=2^0
  o3 : Outport  Port=3  OutDataType=sfix(16)  OutScaling=2^0
  wires:
  Switch1/1 -> o2/1
  ch2/1 -> Switch1/3
  Switch/1 -> o1/1
  ch1/1 -> Switch/3
  Reset/1 -> Discrete-Time Integrator/2
  Constant/1 -> Switch/1, Switch1/1, Switch2/1
  Discrete-Time Integrator/1 -> Switch/2, Switch1/2, Switch2/2
  Constant1/1 -> Discrete-Time Integrator/1
  Switch2/1 -> o3/1
  ch3/1 -> Switch2/3

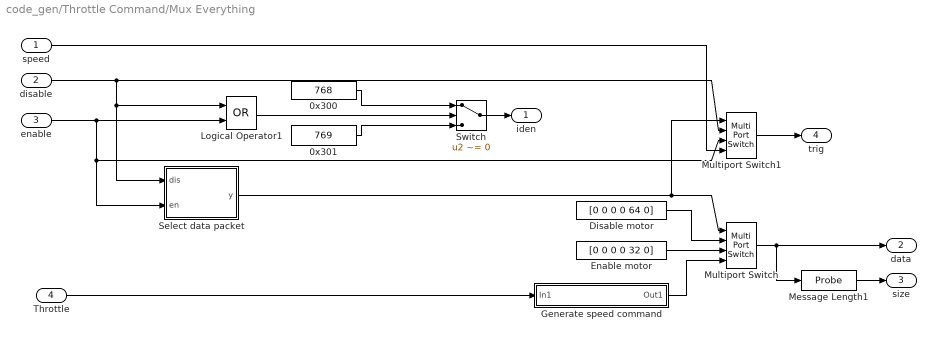
== system code_gen/Throttle Command/Mux Everything ==
  speed : Inport  OutDataType=sfix(16)  OutScaling=2^0
  disable : Inport  Port=2  OutDataType=sfix(16)  OutScaling=2^0
  enable : Inport  Port=3  OutDataType=sfix(16)  OutScaling=2^0
  Throttle : Inport  Port=4  OutDataType=sfix(16)  OutScaling=2^0
  0x300 : Constant  Value=768  OutDataTypeMode=uint32  OutDataType=sfix(16)  OutScaling=2^0  OutDataTypeStr=uint32
  0x301 : Constant  Value=769  OutDataTypeMode=uint32  OutDataType=sfix(16)  OutScaling=2^0  OutDataTypeStr=uint32
  Disable motor : Constant  Value=[0 0 0 0 64 0]  OutDataTypeMode=uint8  OutDataType=sfix(16)  OutScaling=2^0  OutDataTypeStr=uint8
  Enable motor : Constant  Value=[0 0 0 0 32 0]  OutDataTypeMode=uint8  OutDataType=sfix(16)  OutScaling=2^0  OutDataTypeStr=uint8
  Generate speed command : Subsystem
  Logical Operator1 : Logic  Operator=OR  AllPortsSameDT=off  OutDataTypeMode=boolean  OutDataTypeStr=boolean
  Message Length1 : Probe  ProbeSampleTime=off  ProbeComplexSignal=off  ProbeWidthDataType=uint8
  Multiport Switch : MultiPortSwitch  zeroidx=off
  Multiport Switch1 : MultiPortSwitch  zeroidx=off
  Select data packet : Stateflow chart  TreatAsAtomicUnit=on
  Switch : Switch  Criteria=u2 ~= 0
  iden : Outport  OutDataType=sfix(16)  OutScaling=2^0
  data : Outport  Port=2  OutDataType=sfix(16)  OutScaling=2^0
  size : Outport  Port=3  OutDataType=sfix(16)  OutScaling=2^0
  trig : Outport  Port=4  OutDataType=sfix(16)  OutScaling=2^0
  wires:
  Enable motor/1 -> Multiport Switch/3
  Disable motor/1 -> Multiport Switch/2
  Throttle/1 -> Generate speed command/1(In1)
  Multiport Switch/1 -> Message Length1/1, data/1
  Message Length1/1 -> size/1
  0x300/1 -> Switch/1
  0x301/1 -> Switch/3
  Switch/1 -> iden/1
  disable/1 -> Logical Operator1/1, Select data packet/1(dis), Multiport Switch1/2
  enable/1 -> Logical Operator1/2, Select data packet/2(en), Multiport Switch1/3
  Logical Operator1/1 -> Switch/2
  Select data packet/1(y) -> Multiport Switch/1, Multiport Switch1/1
  Generate speed command/1(Out1) -> Multiport Switch/4
  Multiport Switch1/1 -> trig/1
  speed/1 -> Multiport Switch1/4

== system code_gen/Throttle Command/Trigger Events ==
  RC Throttle : Inport  OutDataType=sfix(16)  OutScaling=2^0
  Data Type Conversion3 : DataTypeConversion  OutDataTypeMode=boolean  OutDataType=sfix(16)  OutScaling=2^0  OutDataTypeStr=boolean
  Detect Change : simulink/Logic and Bit Operations/Detect Change  SystemSampleTime=-1  vinit=0
  Detect to/from zero : Subsystem
  Shift Arithmetic : simulink/Logic and Bit Operations/Shift Arithmetic  SystemSampleTime=-1  nBitShiftRight=2  nBinPtShiftRight=0
  Weighted Moving Average : simulink_need_slupdate/Weighted Moving Average  mgainval=[.5 .5]  vinit=0.0  samptime=-1  OutDataTypeStr=Inherit: Inherit via back propagation  OutDataType=sfix(16)  OutScaling=2^-10  DoSatur=off  GainDataType=uint(16)  MatRadixGroup=Best Precision: Matrix-wise  GainScaling=2^-10
  Change Speed : Outport  OutDataType=sfix(16)  OutScaling=2^0
  Disable : Outport  Port=2  OutDataType=sfix(16)  OutScaling=2^0
  Enable : Outport  Port=3  OutDataType=sfix(16)  OutScaling=2^0
  wires:
  RC Throttle/1 -> Shift Arithmetic/1, Detect to/from zero/1(hightime)
  Detect to/from zero/2(Went high) -> Enable/1
  Detect Change/1 -> Data Type Conversion3/1
  Detect to/from zero/1(Went low) -> Disable/1
  Data Type Conversion3/1 -> Change Speed/1
  Weighted Moving Average/1 -> Detect Change/1
  Shift Arithmetic/1 -> Weighted Moving Average/1

== system code_gen/Transmit actuator data/Build HIL sentence ==
  data : Inport
  Bitwise Operator : simulink/Logic and Bit Operations/Bitwise Operator  logicop=XOR  UseBitMask=off  BitMask=bin2dec('11011001')  BitMaskRealWorld=Stored Integer
  Constant : Constant  Value=37  OutDataTypeMode=uint8  OutDataType=fixdt(1, 16)  OutScaling=2^0  OutDataTypeStr=uint8
  Constant1 : Constant  Value=38  OutDataTypeMode=uint8  OutDataType=fixdt(1, 16)  OutScaling=2^0  OutDataTypeStr=uint8
  Constant2 : Constant  Value=94  OutDataTypeMode=uint8  OutDataType=fixdt(1, 16)  OutScaling=2^0  OutDataTypeStr=uint8
  Constant3 : Constant  Value=38  OutDataTypeMode=uint8  OutDataType=fixdt(1, 16)  OutScaling=2^0  OutDataTypeStr=uint8
  Constant4 : Constant  Value=2  OutDataTypeMode=uint8  OutDataType=fixdt(1, 16)  OutScaling=2^0  OutDataTypeStr=uint8
  Mux1 : Mux  Inputs=7
  Mux2 : Mux  Inputs=2
  sent : Outport
  wires:
  data/1 -> Mux1/4, Mux2/2
  Constant/1 -> Mux1/1
  Constant1/1 -> Mux1/2
  Mux1/1 -> sent/1
  Constant4/1 -> Mux1/3, Mux2/1
  Constant2/1 -> Mux1/5
  Constant3/1 -> Mux1/6
  Bitwise Operator/1 -> Mux1/7
  Mux2/1 -> Bitwise Operator/1

== system code_gen/Autonomous Controller/Ballast Command/Calculate Optimal Roll ==
  bearing : Inport  OutDataType=sfix(16)  OutScaling=2^0
  azimuth : Inport  Port=2  OutDataType=sfix(16)  OutScaling=2^0
  zenith : Inport  Port=3  OutDataType=sfix(16)  OutScaling=2^0
  Product : Product  OutDataType=sfix(16)  OutScaling=2^0  RndMeth=Zero
  Subtract : Sum  Inputs=-+  OutDataType=sfix(16)  OutScaling=2^-10
  Trigonometric Function : Trigonometry
  Trigonometric Function1 : Trigonometry
  Trigonometric Function2 : Trigonometry  Operator=atan2
  Trigonometric Function3 : Trigonometry  Operator=cos
  Roll : Outport  OutDataType=sfix(16)  OutScaling=2^0
  wires:
  Trigonometric Function/1 -> Product/2
  Trigonometric Function1/1 -> Product/1
  Product/1 -> Trigonometric Function2/1
  Trigonometric Function3/1 -> Trigonometric Function2/2
  Subtract/1 -> Trigonometric Function1/1
  bearing/1 -> Subtract/1
  zenith/1 -> Trigonometric Function/1, Trigonometric Function3/1
  Trigonometric Function2/1 -> Roll/1
  azimuth/1 -> Subtract/2

== system code_gen/Autonomous Controller/Ballast Command/Map from 313..620 to 1..-1 ==
  In1 : Inport
  Bias : Bias  Bias=-466.5
  Data Type Conversion : DataTypeConversion  OutDataTypeMode=single  OutDataType=fixdt(1, 16)  OutScaling=2^0  OutDataTypeStr=single
  Gain : Gain  Gain=-1/153.5  ParameterDataType=fixdt(1, 16)  ParameterScaling=2^0  OutDataType=fixdt(1, 16)  OutScaling=2^0
  Out1 : Outport
  wires:
  Bias/1 -> Gain/1
  In1/1 -> Data Type Conversion/1
  Gain/1 -> Out1/1
  Data Type Conversion/1 -> Bias/1

== system code_gen/Autonomous Controller/Rudder Command/Map from 313..620 to 1..-1 ==
  In1 : Inport
  Bias : Bias  Bias=-466.5
  Data Type Conversion : DataTypeConversion  OutDataTypeMode=single  OutDataType=fixdt(1, 16)  OutScaling=2^0  OutDataTypeStr=single
  Gain : Gain  Gain=-1/153.5  ParameterDataType=fixdt(1, 16)  ParameterScaling=2^0  OutDataType=fixdt(1, 16)  OutScaling=2^0
  Out1 : Outport
  wires:
  Bias/1 -> Gain/1
  In1/1 -> Data Type Conversion/1
  Gain/1 -> Out1/1
  Data Type Conversion/1 -> Bias/1

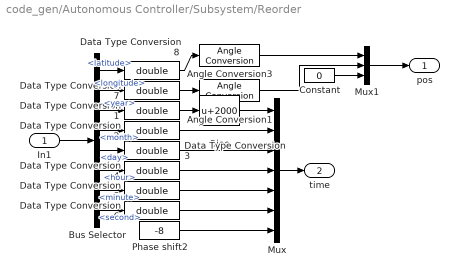
== system code_gen/Autonomous Controller/Subsystem/Reorder ==
  In1 : Inport
  Angle Conversion1 : aerolibconvert2/Angle Conversion  SystemSampleTime=-1  IU=deg  OU=rad
  Angle Conversion3 : aerolibconvert2/Angle Conversion  SystemSampleTime=-1  IU=deg  OU=rad
  Bias : Bias  Bias=2000
  Bus Selector : BusSelector  OutputSignals=latitude,longitude,year,month,day,hour,minute,second
  Constant : Constant  Value=0  OutDataType=fixdt(1, 16)  OutScaling=2^0
  Data Type Conversion{1..8} (8 alike) : DataTypeConversion  OutDataTypeMode=double  OutDataType=fixdt(1, 16)  OutScaling=2^0  OutDataTypeStr=double
  Mux : Mux  Inputs=7
  Mux1 : Mux  Inputs=3
  Phase shift2 : Constant  Value=-8  OutDataType=sfix(16)  OutScaling=2^0
  pos : Outport
  time : Outport  Port=2
  wires:
  Bus Selector/1 -> Data Type Conversion8/1  "<latitude>"
  Bus Selector/2 -> Data Type Conversion7/1  "<longitude>"
  Data Type Conversion1/1 -> Bias/1
  Bias/1 -> Mux/1
  Data Type Conversion2/1 -> Mux/2
  Bus Selector/3 -> Data Type Conversion1/1  "<year>"
  Bus Selector/4 -> Data Type Conversion2/1  "<month>"
  Bus Selector/5 -> Data Type Conversion3/1  "<day>"
  Bus Selector/6 -> Data Type Conversion4/1  "<hour>"
  Bus Selector/7 -> Data Type Conversion5/1  "<minute>"
  Bus Selector/8 -> Data Type Conversion6/1  "<second>"
  Data Type Conversion3/1 -> Mux/3
  Data Type Conversion4/1 -> Mux/4
  Data Type Conversion5/1 -> Mux/5
  Data Type Conversion6/1 -> Mux/6
  Phase shift2/1 -> Mux/7
  In1/1 -> Bus Selector/1
  Mux/1 -> time/1
  Angle Conversion3/1 -> Mux1/1
  Angle Conversion1/1 -> Mux1/2
  Constant/1 -> Mux1/3
  Mux1/1 -> pos/1
  Data Type Conversion7/1 -> Angle Conversion1/1
  Data Type Conversion8/1 -> Angle Conversion3/1

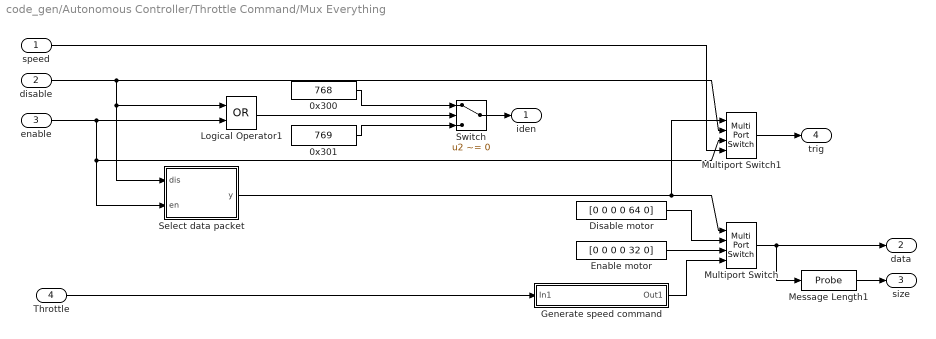
== system code_gen/Autonomous Controller/Throttle Command/Mux Everything ==
  speed : Inport  OutDataType=sfix(16)  OutScaling=2^0
  disable : Inport  Port=2  OutDataType=sfix(16)  OutScaling=2^0
  enable : Inport  Port=3  OutDataType=sfix(16)  OutScaling=2^0
  Throttle : Inport  Port=4  OutDataType=sfix(16)  OutScaling=2^0
  0x300 : Constant  Value=768  OutDataTypeMode=uint32  OutDataType=sfix(16)  OutScaling=2^0  OutDataTypeStr=uint32
  0x301 : Constant  Value=769  OutDataTypeMode=uint32  OutDataType=sfix(16)  OutScaling=2^0  OutDataTypeStr=uint32
  Disable motor : Constant  Value=[0 0 0 0 64 0]  OutDataTypeMode=uint8  OutDataType=sfix(16)  OutScaling=2^0  OutDataTypeStr=uint8
  Enable motor : Constant  Value=[0 0 0 0 32 0]  OutDataTypeMode=uint8  OutDataType=sfix(16)  OutScaling=2^0  OutDataTypeStr=uint8
  Generate speed command : Subsystem
  Logical Operator1 : Logic  Operator=OR  AllPortsSameDT=off  OutDataTypeMode=boolean  OutDataTypeStr=boolean
  Message Length1 : Probe  ProbeSampleTime=off  ProbeComplexSignal=off  ProbeWidthDataType=uint8
  Multiport Switch : MultiPortSwitch  zeroidx=off
  Multiport Switch1 : MultiPortSwitch  zeroidx=off
  Select data packet : Stateflow chart  TreatAsAtomicUnit=on
  Switch : Switch  Criteria=u2 ~= 0
  iden : Outport  OutDataType=sfix(16)  OutScaling=2^0
  data : Outport  Port=2  OutDataType=sfix(16)  OutScaling=2^0
  size : Outport  Port=3  OutDataType=sfix(16)  OutScaling=2^0
  trig : Outport  Port=4  OutDataType=sfix(16)  OutScaling=2^0
  wires:
  speed/1 -> Multiport Switch1/4
  Multiport Switch1/1 -> trig/1
  Generate speed command/1(Out1) -> Multiport Switch/4
  Select data packet/1(y) -> Multiport Switch1/1, Multiport Switch/1
  Logical Operator1/1 -> Switch/2
  enable/1 -> Multiport Switch1/3, Select data packet/2(en), Logical Operator1/2
  disable/1 -> Multiport Switch1/2, Select data packet/1(dis), Logical Operator1/1
  Switch/1 -> iden/1
  0x301/1 -> Switch/3
  0x300/1 -> Switch/1
  Message Length1/1 -> size/1
  Multiport Switch/1 -> data/1, Message Length1/1
  Throttle/1 -> Generate speed command/1(In1)
  Disable motor/1 -> Multiport Switch/2
  Enable motor/1 -> Multiport Switch/3

== system code_gen/Autonomous Controller/Throttle Command/Trigger Events ==
  RC Throttle : Inport  OutDataType=sfix(16)  OutScaling=2^0
  Data Type Conversion3 : DataTypeConversion  OutDataTypeMode=boolean  OutDataType=sfix(16)  OutScaling=2^0  OutDataTypeStr=boolean
  Detect Change : simulink/Logic and Bit Operations/Detect Change  SystemSampleTime=-1  vinit=0
  Detect to/from zero : Subsystem
  Shift Arithmetic : simulink/Logic and Bit Operations/Shift Arithmetic  SystemSampleTime=-1  nBitShiftRight=2  nBinPtShiftRight=0
  Weighted Moving Average : simulink_need_slupdate/Weighted Moving Average  mgainval=[.5 .5]  vinit=0.0  samptime=-1  OutDataTypeStr=Inherit: Inherit via back propagation  OutDataType=sfix(16)  OutScaling=2^-10  DoSatur=off  GainDataType=uint(16)  MatRadixGroup=Best Precision: Matrix-wise  GainScaling=2^-10
  Change Speed : Outport  OutDataType=sfix(16)  OutScaling=2^0
  Disable : Outport  Port=2  OutDataType=sfix(16)  OutScaling=2^0
  Enable : Outport  Port=3  OutDataType=sfix(16)  OutScaling=2^0
  wires:
  Shift Arithmetic/1 -> Weighted Moving Average/1
  Weighted Moving Average/1 -> Detect Change/1
  Data Type Conversion3/1 -> Change Speed/1
  Detect to/from zero/1(Went low) -> Disable/1
  Detect Change/1 -> Data Type Conversion3/1
  Detect to/from zero/2(Went high) -> Enable/1
  RC Throttle/1 -> Detect to/from zero/1(hightime), Shift Arithmetic/1

== system code_gen/Propulsion Outputs/To Drive Motor/C-function Call ==
  parameters : Inport  OutDataType=sfix(16)  OutScaling=2^0
  Enable : EnablePort
  ECAN1 Transmit [ecanFunctions.c] : dsPICdrivers/OTHERS/C Function Call  Tag=dsPIC_dsPIC_CFunctionCall  fctName='ecan1_buffered_transmit_matlab'  INPUT_SIZE=8  INPUT1=uint16  INPUT2=--  INPUT3=--  OUTPUT_SIZE=1  OUTPUT1=--  SampleTime=c_func_sample_time  InputType=[ 4 ]  OutputType=[ ]  FctDeclaration=extern void ecan1_buffered_transmit_matlab(uint16_T* u1);  FctCall=ecan1_buffered_transmit_matlab(*%u1);  OrderingInOutPopup=None
  wires:
  parameters/1 -> ECAN1 Transmit [ecanFunctions.c]/1
